simulink library "NNodeTether_cl"  (R2022a)
settings: Solver=VariableStepAuto  StartTime=0.0  StopTime=10.0  RelTol=1e-3
values from neighbouring files (symbols this model uses):
  numNodes = thr(1).numNodes    [NNodeTether_init.m]    (also in tetherFaired_init.m = dimInfo.numNodes)
undefined symbols (not defined in the file or in its folder): fluidDensity, gravity, thrStructure
libraries: nodeDragForce_ul x1, nodeNetBuoyForce_ul x1, nodePosToLinkPos_ul x1, nodeSpringDamperForce_ul x1, thrNodeMass_ul x1
settings Model: Creator=mcobb  LastModifiedBy=lhill8
settings SolverCC: AlgebraicLoopSolver=TrustRegion
settings DebuggingCC: UnconnectedInputMsg=warning  UnconnectedOutputMsg=warning  UnconnectedLineMsg=warning  SFMachineParentedDataDiag=warning  ArithmeticOperatorsInVariantConditions=warning
settings SFSimCC: CustomCodeUndefinedFunction=UseInterfaceOnly

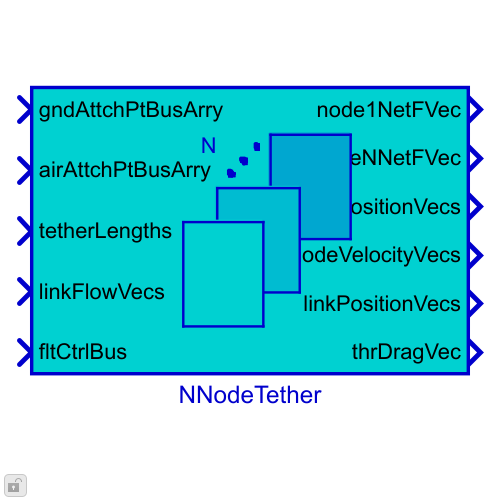
[thumbnail: Simulink's stored preview of the top-level diagram]
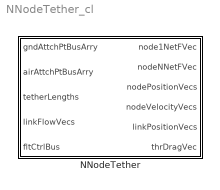
== system NNodeTether_cl ==
  NNodeTether : Subsystem  VariantControl=NNodeTether  mask{thr=thrStructure, flowDensity=fluidDensity, gravity=gravity}
      mask prompts: thr "Tether Structure"; flowDensity "Fluid Density"; gravity "Gravitational Acceleration"

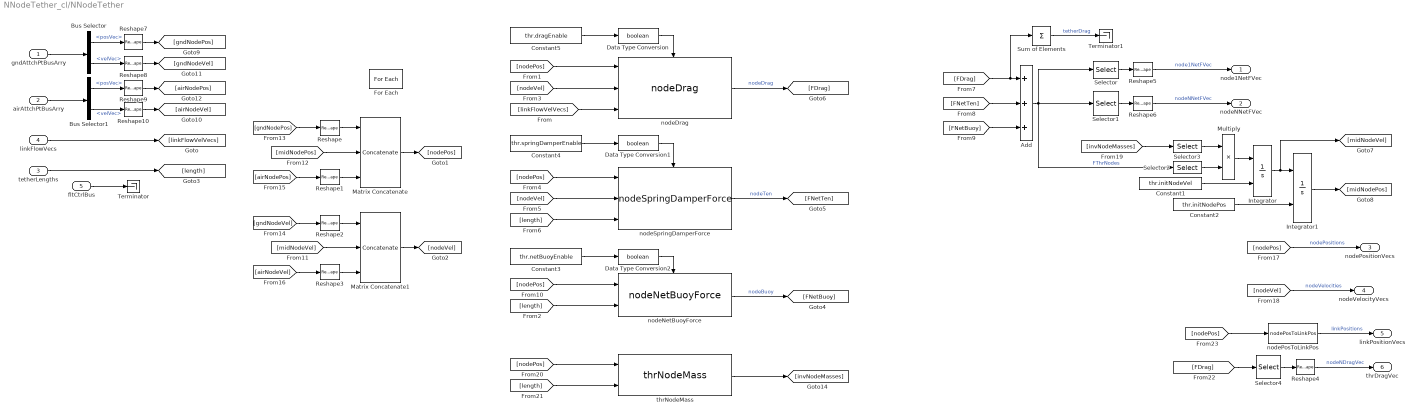
== system NNodeTether_cl/NNodeTether ==
  gndAttchPtBusArry : Inport  OutDataTypeStr=Bus: thrAttachPtKinematicsBus  Partition=on  PartitionDimension=1  PartitionWidth=1  PartitionOffset=0
  airAttchPtBusArry : Inport  Port=2  OutDataTypeStr=Bus: thrAttachPtKinematicsBus  Partition=on  PartitionDimension=1  PartitionWidth=1  PartitionOffset=0
  tetherLengths : Inport  Port=3  Partition=on  PartitionDimension=1  PartitionWidth=1  PartitionOffset=0
  linkFlowVecs : Inport  Port=4  Partition=on  PartitionDimension=3  PartitionWidth=1  PartitionOffset=0
  fltCtrlBus : Inport  Port=5
  Add : Sum  Inputs=3
  Bus Selector : BusSelector  OutputSignals=posVec,velVec
  Bus Selector1 : BusSelector  OutputSignals=posVec,velVec
  Constant1 : Constant  Value=thr.initNodeVel
  Constant2 : Constant  Value=thr.initNodePos
  Constant3 : Constant  Value=thr.netBuoyEnable
  Constant4 : Constant  Value=thr.springDamperEnable
  Constant5 : Constant  Value=thr.dragEnable
  Data Type Conversion : DataTypeConversion  OutDataTypeStr=boolean  SaturateOnIntegerOverflow=off  RndMeth=Floor
  Data Type Conversion1 : DataTypeConversion  OutDataTypeStr=boolean  SaturateOnIntegerOverflow=off  RndMeth=Floor
  Data Type Conversion2 : DataTypeConversion  OutDataTypeStr=boolean  SaturateOnIntegerOverflow=off  RndMeth=Floor
  For Each : ForEach  DisableCoverage=on  IterateSubsysMaskParameter=on,off,off  SubsysMaskParameterIterationDimension=2,1,1  SubsysMaskParameterIterationStepSize=1,1,1
  Integrator : Integrator  InitialConditionSource=external
  Integrator1 : Integrator  InitialConditionSource=external
  Matrix Concatenate : Concatenate  NumInputs=3  Mode=Multidimensional array  ConcatenateDimension=2
  Matrix Concatenate1 : Concatenate  NumInputs=3  Mode=Multidimensional array  ConcatenateDimension=2
  Multiply : Product
  Reshape{,1..10} (11 alike) : Reshape  OutputDimensionality=Column vector (2-D)
  Selector : Selector  NumberOfDimensions=2  InputPortWidth=3  IndexOptions=Select all,Index vector (dialog)  Indices=[1 3],1  OutputSizes=1,1
  Selector1 : Selector  NumberOfDimensions=2  InputPortWidth=3  IndexOptions=Select all,Starting index (dialog)  Indices=[1 3],numNodes  OutputSizes=1,1
  Selector2 : Selector  NumberOfDimensions=2  InputPortWidth=3  IndexOptions=Select all,Index vector (dialog)  Indices=[1 3],2:numNodes-1  OutputSizes=1,1
  Selector3 : Selector  NumberOfDimensions=2  InputPortWidth=3  IndexOptions=Select all,Index vector (dialog)  Indices=[1 3],2:numNodes-1  OutputSizes=1,1
  Selector4 : Selector  NumberOfDimensions=2  InputPortWidth=3  IndexOptions=Select all,Starting index (dialog)  Indices=[1 3],numNodes  OutputSizes=1,1
  Sum of Elements : Sum  Inputs=+  CollapseMode=Specified dimension  CollapseDim=2
  Terminator : Terminator
  Terminator1 : Terminator
  nodeDrag : nodeDragForce_ul/nodeDrag  flowDensity=flowDensity  thrDiam=thr.diameter  dragCoeff=thr.dragCoeff
  nodeNetBuoyForce : nodeNetBuoyForce_ul/nodeNetBuoyForce  fluidDensity=flowDensity  tetherDensity=thr.density  diameter=thr.diameter  gravity=gravity
  nodePosToLinkPos : nodePosToLinkPos_ul/nodePosToLinkPos  SystemSampleTime=-1  VariantActivationTime=update diagram  Latency=0  AutoFrameSizeCalculation=off
  nodeSpringDamperForce : nodeSpringDamperForce_ul/nodeSpringDamperForce  mass=thr.vehicleMass  zeta=thr.dampingRatio  diameter=thr.diameter  youngsMod=thr.youngsMod
  thrNodeMass : thrNodeMass_ul/thrNodeMass  tetherDensity=thr.density  diameter=thr.diameter
  node1NetFVec : Outport  ConcatenationDimension=3  VectorParamsAs1DForOutWhenUnconnected=off
  nodeNNetFVec : Outport  Port=2  ConcatenationDimension=3  VectorParamsAs1DForOutWhenUnconnected=off
  nodePositionVecs : Outport  Port=3  ConcatenationDimension=3  VectorParamsAs1DForOutWhenUnconnected=off
  nodeVelocityVecs : Outport  Port=4  ConcatenationDimension=3  VectorParamsAs1DForOutWhenUnconnected=off
  linkPositionVecs : Outport  Port=5  ConcatenationDimension=3  VectorParamsAs1DForOutWhenUnconnected=off
  thrDragVec : Outport  Port=6  ConcatenationDimension=3  VectorParamsAs1DForOutWhenUnconnected=off
  wires:
  [nodePos] -> nodeNetBuoyForce/1
  Selector1/1 -> Reshape6/1
  Add/1 -> Selector1/1, Selector2/1, Selector/1  "FThrNodes"
  Selector/1 -> Reshape5/1
  [FNetBuoy] -> Add/3
  [FDrag] -> Sum of Elements/1, Add/1
  [FNetTen] -> Add/2
  nodeDrag/1 -> [FDrag]  "nodeDrag"
  nodeSpringDamperForce/1 -> [FNetTen]  "nodeTen"
  nodeNetBuoyForce/1 -> [FNetBuoy]  "nodeBuoy"
  [length] -> nodeSpringDamperForce/3
  [nodePos] -> nodeSpringDamperForce/1
  [nodeVel] -> nodeSpringDamperForce/2
  [nodeVel] -> nodeDrag/2
  [length] -> nodeNetBuoyForce/2
  [nodePos] -> nodeDrag/1
  [linkFlowVelVecs] -> nodeDrag/3
  Reshape2/1 -> Matrix Concatenate1/1
  Reshape3/1 -> Matrix Concatenate1/3
  Reshape1/1 -> Matrix Concatenate/3
  Reshape/1 -> Matrix Concatenate/1
  [airNodeVel] -> Reshape3/1
  [airNodePos] -> Reshape1/1
  [gndNodeVel] -> Reshape2/1
  [gndNodePos] -> Reshape/1
  Selector2/1 -> Multiply/2
  Integrator/1 -> Integrator1/1, [midNodeVel]
  Integrator1/1 -> [midNodePos]
  [midNodeVel] -> Matrix Concatenate1/2
  [midNodePos] -> Matrix Concatenate/2
  Matrix Concatenate/1 -> [nodePos]
  Reshape10/1 -> [airNodeVel]
  airAttchPtBusArry/1 -> Bus Selector1/1
  Bus Selector/2 -> Reshape8/1  "<velVec>"
  gndAttchPtBusArry/1 -> Bus Selector/1
  tetherLengths/1 -> [length]
  Bus Selector1/1 -> Reshape9/1  "<posVec>"
  Reshape9/1 -> [airNodePos]
  Reshape7/1 -> [gndNodePos]
  Bus Selector1/2 -> Reshape10/1  "<velVec>"
  Bus Selector/1 -> Reshape7/1  "<posVec>"
  Reshape8/1 -> [gndNodeVel]
  Multiply/1 -> Integrator/1
  Data Type Conversion2/1 -> nodeNetBuoyForce/Enable
  Constant3/1 -> Data Type Conversion2/1
  Constant4/1 -> Data Type Conversion1/1
  Data Type Conversion1/1 -> nodeSpringDamperForce/Enable
  Constant5/1 -> Data Type Conversion/1
  Data Type Conversion/1 -> nodeDrag/Enable
  Constant1/1 -> Integrator/2
  Constant2/1 -> Integrator1/2
  Selector3/1 -> Multiply/1
  [invNodeMasses] -> Selector3/1
  Matrix Concatenate1/1 -> [nodeVel]
  [nodePos] -> thrNodeMass/1
  [length] -> thrNodeMass/2
  thrNodeMass/1 -> [invNodeMasses]
  linkFlowVecs/1 -> [linkFlowVelVecs]
  [nodePos] -> nodePosToLinkPos/1
  Reshape5/1 -> node1NetFVec/1  "node1NetFVec"
  Reshape6/1 -> nodeNNetFVec/1  "nodeNNetFVec"
  [nodePos] -> nodePositionVecs/1  "nodePositions"
  [nodeVel] -> nodeVelocityVecs/1  "nodeVelocities"
  nodePosToLinkPos/1 -> linkPositionVecs/1  "linkPositions"
  Selector4/1 -> Reshape4/1
  [FDrag] -> Selector4/1
  Reshape4/1 -> thrDragVec/1  "nodeNDragVec"
  fltCtrlBus/1 -> Terminator/1
  Sum of Elements/1 -> Terminator1/1  "tetherDrag"
